simulink model "RCLparallel_sim"  (R2024a)
settings: Solver=VariableStepAuto  StartTime=0.0  StopTime=t_sim  RelTol=1e-3
values from neighbouring files (symbols this model uses):
  C = 0.25    [RLCparallel.m]
  L = 0.5    [RLCparallel.m]
  R = 3    [RLCparallel.m]
settings Model: Creator=lorenzo  LastModifiedBy=lorenzo

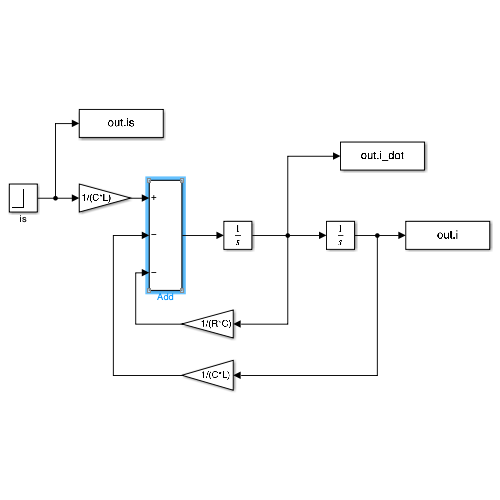
[thumbnail: Simulink's stored preview of the top-level diagram]
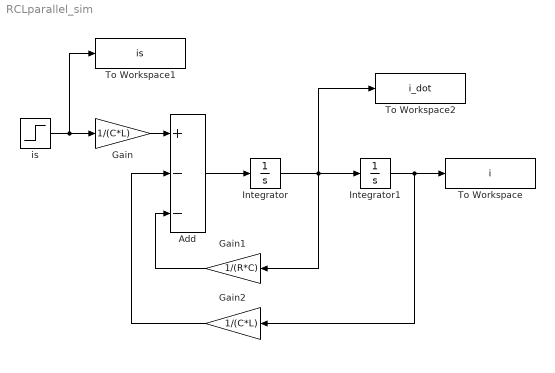
== system RCLparallel_sim ==
  Add : Sum  Inputs=+--
  Gain : Gain  Gain=1/(C*L)
  Gain1 : Gain  Gain=1/(R*C)
  Gain2 : Gain  Gain=1/(C*L)
  Integrator : Integrator
  Integrator1 : Integrator
  To Workspace : ToWorkspace  VariableName=i  SaveFormat=Timeseries  SampleTime=-1
  To Workspace1 : ToWorkspace  VariableName=is  SaveFormat=Timeseries  SampleTime=-1
  To Workspace2 : ToWorkspace  VariableName=i_dot  SaveFormat=Timeseries  SampleTime=-1
  is : Step  Time=0  After=5  SampleTime=0
  wires:
  is/1 -> Gain/1, To Workspace1/1
  Gain/1 -> Add/1
  Add/1 -> Integrator/1
  Integrator/1 -> To Workspace2/1, Gain1/1, Integrator1/1
  Gain1/1 -> Add/3
  Integrator1/1 -> To Workspace/1, Gain2/1
  Gain2/1 -> Add/2
